simulink model "Heartbridge"  (R2024b)
settings: Solver=ode45  StartTime=0.0  StopTime=10.0  MaxStep=0.5*Ts  RelTol=1e-3
values from neighbouring files (symbols this model uses):
  accel_limit = -1    [simulinkSetup.m]
  b = 0    [simulinkSetup.m]
  eta_ball = 0.8    [simulinkSetup.m]
  iLimit = 10    [simulinkSetup.m]
  iRateLimit = -1    [simulinkSetup.m]
  J_ball = (pi*rho_ball*length_ball*D_ball^4)/32    (= 2.93733050036e-07)    [simulinkSetup.m]
  J_m = 2.367e-6    (= 2.367e-06)    [simulinkSetup.m]
  k = 0    [simulinkSetup.m]
  K_torque = (3/2)*(1/sqrt(3))*(60/(2*pi))/K_v    [simulinkSetup.m]
  m_ball = 2    [simulinkSetup.m]
  p_ball = L_ball/(2*pi)    (= 0.00202126777727)    [simulinkSetup.m]
  pid_dq_hz = 100    [simulinkSetup.m]
  servo_max_current = 120    [simulinkSetup.m]
  tau_d = 1.5*Ts    (= 0.0001)    [simulinkSetup.m]
  tau_max_ball = F_max*L_ball/(2*pi*eta_ball)    (= 1.26329236079)    [simulinkSetup.m]
  Ts = 1/servo_pwm_rate_hz    (= 6.66666666667e-05)    [simulinkSetup.m]
  vel_limit = -1    [simulinkSetup.m]
  w_n_pll = 2*pi*f_pll/2.48    (= 1013.41698503)    [simulinkSetup.m]
  zeta_pll = 1    [simulinkSetup.m]
undefined symbols (not defined in the file or in its folder): DiscIntNeverNeededParam
libraries: simulink x2
settings Model: Creator=danie  LastModifiedBy=Daniel G

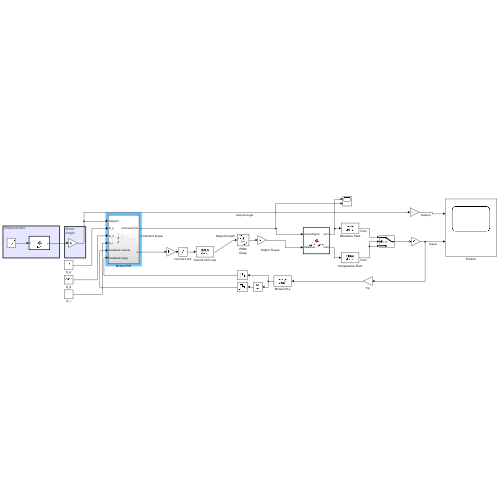
[thumbnail: Simulink's stored preview of the top-level diagram]
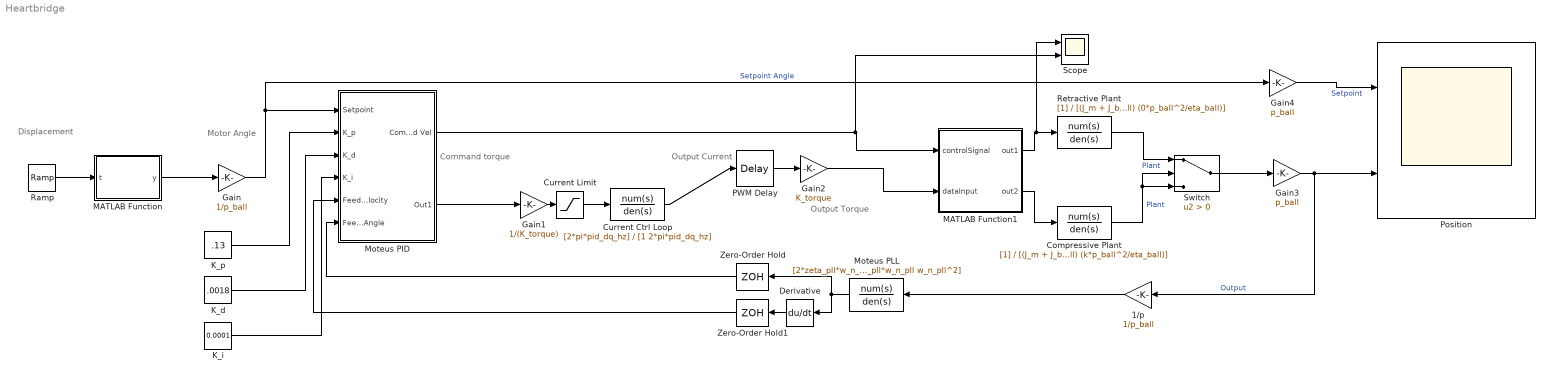
== system Heartbridge ==
  note: Output Torque
  note: Output Current
  note: Command torque
  note: Motor
      | Angle
  note: Displacement
  1/p : Gain  Gain=1/p_ball
  Compressive Plant : TransferFcn  Denominator=[(J_m + J_ball + m_ball*p_ball^2/eta_ball) (b*p_ball^2/eta_ball) (k*p_ball^2/eta_ball)]
  Current Ctrl Loop : TransferFcn  Numerator=[2*pi*pid_dq_hz]  Denominator=[1 2*pi*pid_dq_hz]
  Current Limit : Saturate  UpperLimit=servo_max_current  LowerLimit=-servo_max_current
  Derivative : Derivative
  Gain : Gain  Gain=1/p_ball
  Gain1 : Gain  Gain=1/(K_torque)
  Gain2 : Gain  Gain=K_torque
  Gain3 : Gain  Gain=p_ball
  Gain4 : Gain  Gain=p_ball
  K_d : Constant  Value=.0018
  K_i : Constant  Value=0.0001
  K_p : Constant  Value=.13
  MATLAB Function : MATLAB Function  TreatAsAtomicUnit=on
  MATLAB Function1 : MATLAB Function  TreatAsAtomicUnit=on
  Moteus PID : Subsystem
  Moteus PLL : TransferFcn  Numerator=[2*zeta_pll*w_n_pll w_n_pll^2]  Denominator=[1 2*zeta_pll*w_n_pll w_n_pll^2]
  PWM Delay : TransportDelay  DelayTime=tau_d
  Position : Scope  NumInputPorts=2
  Ramp : simulink/Sources/Ramp  slope=1  start=0  InitialOutput=0
  Retractive Plant : TransferFcn  Denominator=[(J_m + J_ball + m_ball*p_ball^2/eta_ball) (0*p_ball^2/eta_ball) (0*p_ball^2/eta_ball)]
  Scope : Scope  NumInputPorts=2
  Switch : Switch  Criteria=u2 > Threshold  SaturateOnIntegerOverflow=off  InputSameDT=off
  Zero-Order Hold : ZeroOrderHold  SampleTime=Ts
  Zero-Order Hold1 : ZeroOrderHold  SampleTime=Ts
  wires:
  Ramp/1 -> MATLAB Function/1(t)
  MATLAB Function/1(y) -> Gain/1
  Gain/1 -> Gain4/1, Moteus PID/1(Setpoint)  "Setpoint Angle"
  K_p/1 -> Moteus PID/2(K_p)
  K_d/1 -> Moteus PID/3(K_d)
  K_i/1 -> Moteus PID/4(K_i)
  Moteus PID/2(Out1) -> Gain1/1
  Gain1/1 -> Current Limit/1
  Current Limit/1 -> Current Ctrl Loop/1
  Current Ctrl Loop/1 -> PWM Delay/1
  PWM Delay/1 -> Gain2/1
  Moteus PLL/1 -> Zero-Order Hold/1, Derivative/1
  Derivative/1 -> Zero-Order Hold1/1
  Zero-Order Hold1/1 -> Moteus PID/5(Feedback Velocity)
  Zero-Order Hold/1 -> Moteus PID/6(Feedback Angle)
  Gain3/1 -> Position/2, 1/p/1  "Output"
  1/p/1 -> Moteus PLL/1
  Gain4/1 -> Position/1  "Setpoint"
  Gain2/1 -> MATLAB Function1/2(dataInput)
  MATLAB Function1/2(out2) -> Compressive Plant/1
  MATLAB Function1/1(out1) -> Scope/1, Retractive Plant/1
  Switch/1 -> Gain3/1
  Compressive Plant/1 -> Switch/3, Switch/2  "Plant"
  Retractive Plant/1 -> Switch/1  "Plant"
  Moteus PID/1(Command Vel) -> Scope/2, MATLAB Function1/1(controlSignal)

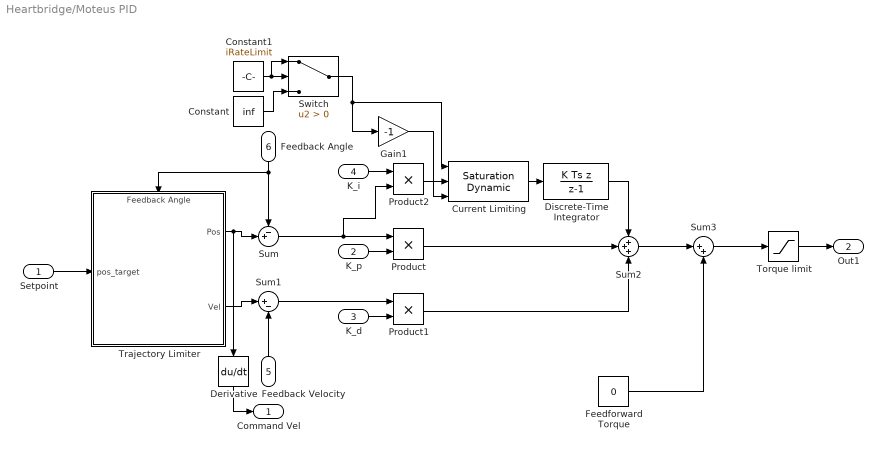
== system Heartbridge/Moteus PID ==
  Setpoint : Inport
  K_p : Inport  Port=2
  K_d : Inport  Port=3
  K_i : Inport  Port=4
  Feedback Velocity : Inport  Port=5
  Feedback Angle : Inport  Port=6
  Constant : Constant  Value=inf
  Constant1 : Constant  Value=iRateLimit
  Current Limiting : simulink/Discontinuities/Saturation Dynamic  OutMin=[]  OutMax=[]  OutDataTypeStr=Inherit: Same as second input  OutDataType=fixdt(1, 16)  OutScaling=2^-10  DoSatur=off
  Derivative : Derivative
  Discrete-Time Integrator : DiscreteIntegrator  IntegratorMethod=Integration: Backward Euler  SampleTime=-1  LimitOutput=on  UpperSaturationLimit=iLimit  LowerSaturationLimit=-iLimit  ICPrevOutput=DiscIntNeverNeededParam  ICPrevScaledInput=DiscIntNeverNeededParam
  Feedforward Torque : Constant  Value=0
  Gain1 : Gain  Gain=-1
  Product : Product
  Product1 : Product
  Product2 : Product
  Sum : Sum  Inputs=-+|
  Sum1 : Sum  Inputs=|+-
  Sum2 : Sum  Inputs=+++
  Sum3 : Sum  Inputs=|++
  Switch : Switch  Criteria=u2 > Threshold  SaturateOnIntegerOverflow=off  InputSameDT=off
  Torque limit : Saturate  UpperLimit=tau_max_ball  LowerLimit=-tau_max_ball
  Trajectory Limiter : Subsystem
      settings: PortSchema="{\"entries\":[{\"content\":{\"sides\":[{\"content\":{\"connectorIds\":[\"In1\"]},\"type\":\"ConnectorPlacement.EquallySpacedRectSide\",\"uuid\":\"61548264-7453-4a29-bd66-f960738fac7f\"},{\"content\":{\"connectorIds\":[\"Out1\",\"Out2\"],\"side\":\"RIGHT\"},\"type\":\"ConnectorPlacement.EquallySpacedRectSide\",\"uuid\":\"f716a689-e738-4715-bb87-0b02ddc273b1\"},{\"content\":{\"connectorIds\":[\"In2\"],\"side\":\"TOP\"},\"type\":\"ConnectorPlacement.EquallySpacedRectSide\",\"uuid\":\"a8aad9a9-d98c-4bd5-94ec-230b36f09c6d\"}]},\"type\":\"ConnectorPlacement.EquallySpacedConnector\",\"uuid\":\"a20a297a-1ecc-4216-a539-303763b08d57\"}],\"packageUris\":[\"http://schema.mathworks.com/mf0/Connector/R2020b\"],\"version\":\"1.0\"}"
  Command Vel : Outport
  Out1 : Outport  Port=2
  wires:
  Feedback Angle/1 -> Trajectory Limiter/2(Feedback Angle), Sum/1
  Feedback Velocity/1 -> Sum1/2
  K_p/1 -> Product/2
  K_d/1 -> Product1/2
  Sum1/1 -> Product1/1
  Sum/1 -> Product2/2, Product/1
  Product/1 -> Sum2/2
  Product1/1 -> Sum2/3
  Constant1/1 -> Switch/1, Switch/2
  Constant/1 -> Switch/3
  Switch/1 -> Gain1/1, Current Limiting/1
  Gain1/1 -> Current Limiting/3
  Sum2/1 -> Sum3/1
  Feedforward Torque/1 -> Sum3/2
  Sum3/1 -> Torque limit/1
  Torque limit/1 -> Out1/1
  K_i/1 -> Product2/1
  Product2/1 -> Current Limiting/2
  Current Limiting/1 -> Discrete-Time Integrator/1
  Discrete-Time Integrator/1 -> Sum2/1
  Setpoint/1 -> Trajectory Limiter/1(pos_target)
  Trajectory Limiter/1(Pos) -> Derivative/1, Sum/2
  Trajectory Limiter/2(Vel) -> Sum1/1
  Derivative/1 -> Command Vel/1

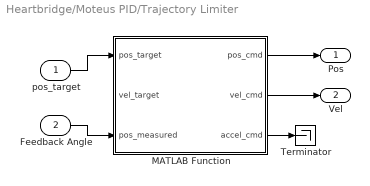
== system Heartbridge/Moteus PID/Trajectory Limiter ==
  pos_target : Inport
  Feedback Angle : Inport  Port=2
  MATLAB Function : MATLAB Function  TreatAsAtomicUnit=on
  Terminator : Terminator
  Pos : Outport
  Vel : Outport  Port=2
  wires:
  MATLAB Function/3(accel_cmd) -> Terminator/1
  MATLAB Function/2(vel_cmd) -> Vel/1
  MATLAB Function/1(pos_cmd) -> Pos/1
  pos_target/1 -> MATLAB Function/1(pos_target)
  Feedback Angle/1 -> MATLAB Function/3(pos_measured)

== matlab function Heartbridge/Moteus PID/Trajectory Limiter/MATLAB Function ==
  settings: updateMethod=DISCRETE  sampleTime=Ts
  data: pos_target input; vel_target input; pos_cmd output; pos_measured input; vel_cmd output; accel_cmd output; Ts parameter; vel_limit parameter; accel_limit parameter
function [pos_cmd, vel_cmd, accel_cmd] = moteus_trajectory_limiter( ...
        pos_target, vel_target, pos_measured, Ts, vel_limit, accel_limit)
% moteus trajectory limiter (BldcServoPosition::UpdateCommand / UpdateTrajectory)
% Negative or NaN limits mean "disabled", as in the firmware.
%   pos_target  : commanded position [rad]
%   vel_target  : commanded velocity sent with the position [rad/s]
%   pos_measured: measured position, used only on the first call [rad]

  persistent pos_state vel_state is_done last_target
  accel_on = isfinite(accel_limit) && accel_limit >= 0;
  vel_on   = isfinite(vel_limit)   && vel_limit   >= 0;

  % ---- Both limits off: pass the command straight through ----
  if ~accel_on && ~vel_on
    pos_state = pos_target;  vel_state = vel_target;
    pos_cmd = pos_target;  vel_cmd = vel_target;  accel_cmd = 0;
    return;
  end

  if isempty(pos_state)
    pos_state = pos_measured;  vel_state = 0;
    is_done = false;  last_target = pos_target;
  end
  if pos_target ~= last_target
    is_done = false;  last_target = pos_target;
  end
  if is_done
    pos_cmd = pos_state;  vel_cmd = 0;  accel_cmd = 0;
    return;
  end

  pos_remaining = pos_target - pos_state;
  vel_start     = vel_state;
  speed_start   = abs(vel_start);

  % ---- Velocity limit only: move at constant +/- vel_limit ----
  if ~accel_on
    vel_state = sign(pos_remaining) * vel_limit;
    if abs(pos_remaining) <= vel_limit * Ts        % this step reaches the target
      pos_state = pos_target;  vel_state = 0;  is_done = true;
    else
      pos_state = pos_state + vel_state * Ts;
    end
    pos_cmd = pos_state;  vel_cmd = vel_state;  accel_cmd = 0;
    return;
  end

  % ---- Acceleration limit (velocity limit inf if unset) ----
  if ~vel_on, vel_limit = inf; end

  if speed_start > vel_limit
    accel = -sign(vel_start) * accel_limit;
  elseif vel_start * pos_remaining >= 0 && pos_remaining ~= 0
    stopping_distance      = vel_start^2 / (2 * accel_limit);
    speed_next             = speed_start + accel_limit * Ts;
    remaining_after_step   = abs(pos_remaining) - (speed_start + speed_next) / 2 * Ts;
    stopping_distance_next = speed_next^2 / (2 * accel_limit);
    if abs(pos_remaining) > stopping_distance && remaining_after_step >= stopping_distance_next
      accel = (speed_start < vel_limit) * sign(pos_remaining) * accel_limit;
    else
      accel = -sign(vel_start) * min(accel_limit, vel_start^2 / (2 * abs(pos_remaining)));
    end
  else
    accel = -sign(vel_start) * accel_limit;
  end

  vel_state = vel_start + accel * Ts;
  speed_end = abs(vel_state);
  if min(speed_start, speed_end) < vel_limit && max(speed_start, speed_end) > vel_limit
    vel_state = sign(vel_state) * vel_limit;  accel = 0;
  end
  if accel ~= 0
    pos_state = pos_state + (vel_start + vel_state) / 2 * Ts;
  else
    pos_state = pos_state + vel_state * Ts;
  end

  vel_crossed_zero = min(vel_start, vel_state) <= 0 && max(vel_start, vel_state) >= 0;
  vel_near_zero    = abs(vel_state) < accel_limit * Ts / 2;
  pos_near_target  = abs(pos_remaining) <= abs(vel_state) * 10 * Ts;
  if (vel_crossed_zero || vel_near_zero) && pos_near_target
    vel_state = 0;  accel = 0;  is_done = true;
  end

  pos_cmd = pos_state;  vel_cmd = vel_state;  accel_cmd = accel;
end

== matlab function Heartbridge/MATLAB Function ==
  data: t input; y output
function y = fcn(t)
    time = mod(t, .56);
    
    if (time <= .12)
        y = 0;
    elseif (time <= .24)
        y = (-41.6666667*(time - .12))*1e-2;
    elseif (time <= .323)
        y = -5e-2;
    else
        y = (21.0965609*(time - .323) - 5)*1e-2;
    end
end

== matlab function Heartbridge/MATLAB Function1 ==
  data: controlSignal input; out1 output; dataInput input; out2 output
function [out1, out2] = routeSignal(controlSignal, dataInput)
    % Initialize default/idle values for all outputs
    out1 = 0; 
    out2 = 0;

    % Route the active signal based on condition
    if controlSignal > 0
        out1 = dataInput;
    else
        out2 = dataInput;
    end
end
